simulink model "untitled"  (R2023a)
settings: Solver=VariableStepAuto  StartTime=0.0  StopTime=10.0  RelTol=1e-3
settings Model: Creator=Ljubomir  LastModifiedBy=Ljubomir

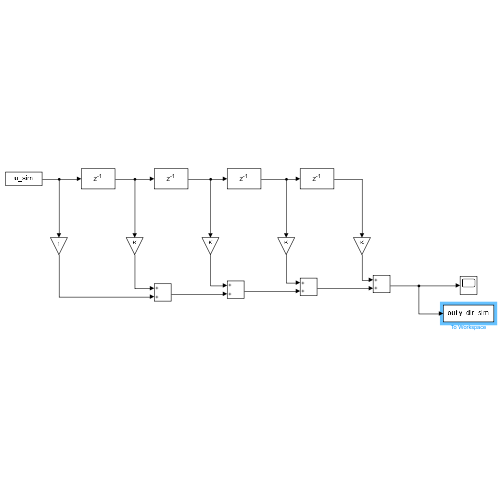
[thumbnail: Simulink's stored preview of the top-level diagram]
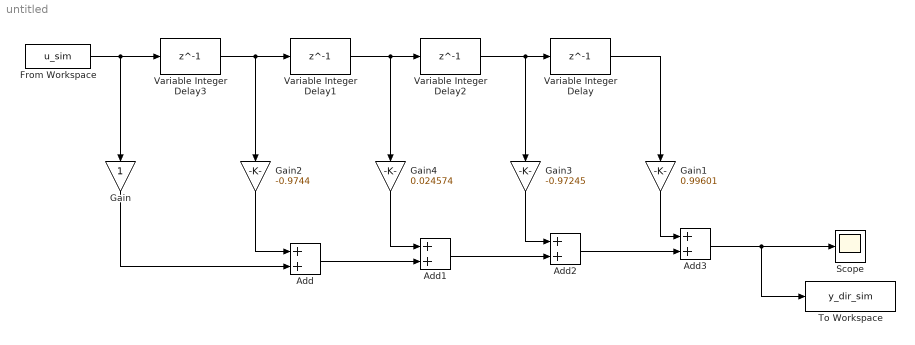
== system untitled ==
  Add{,1..3} (4 alike) : Sum
  From Workspace : FromWorkspace  VariableName=u_sim
  Gain : Gain
  Gain1 : Gain  Gain=0.99601
  Gain2 : Gain  Gain=-0.9744
  Gain3 : Gain  Gain=-0.97245
  Gain4 : Gain  Gain=0.024574
  Scope : Scope
  To Workspace : ToWorkspace  VariableName=y_dir_sim  SampleTime=-1
  Variable Integer Delay{,1..3} (4 alike) : Delay  DelayLength=1
  wires:
  From Workspace/1 -> Gain/1, Variable Integer Delay3/1
  Variable Integer Delay3/1 -> Gain2/1, Variable Integer Delay1/1
  Variable Integer Delay1/1 -> Gain4/1, Variable Integer Delay2/1
  Variable Integer Delay2/1 -> Gain3/1, Variable Integer Delay/1
  Variable Integer Delay/1 -> Gain1/1
  Gain/1 -> Add/2
  Gain2/1 -> Add/1
  Add/1 -> Add1/2
  Gain4/1 -> Add1/1
  Add1/1 -> Add2/2
  Gain3/1 -> Add2/1
  Add2/1 -> Add3/2
  Gain1/1 -> Add3/1
  Add3/1 -> To Workspace/1, Scope/1
